simulink model "lccde2"  (Simulink 8.3)
settings: Solver=ode3  StartTime=0.0  StopTime=10.0  FixedStep=0.01  RelTol=1e-3
libraries: simulink x1
settings Model: Creator=Administrator  LastModifiedBy=Administrator
settings DataIOCC: SignalLoggingSaveFormat=Dataset
settings DebuggingCC: UnderspecifiedInitializationDetection=Simplified  StateNameClashWarn=none
settings GRTTargetCC: CombineOutputUpdateFcns=on  GRTInterface=off

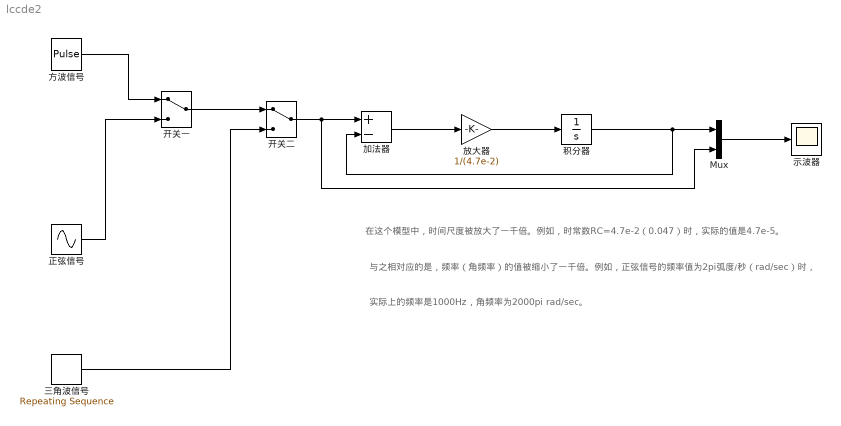
== system lccde2 ==
  note: 实际上的频率是1000Hz，角频率为2000pi rad/sec。
  note: 与之相对应的是，频率（角频率）的值被缩小了一千倍。例如，正弦信号的频率值为2pi弧度/秒（rad/sec）时，
  note: 在这个模型中，时间尺度被放大了一千倍。例如，时常数RC=4.7e-2（0.047）时，实际的值是4.7e-5。
  Mux : Mux  Inputs=2
  三角波信号 : simulink/Sources/Repeating Sequence  rep_seq_t=[0 0.5 1]  rep_seq_y=[0 2 0]
  加法器 : Sum  Inputs=+-
  开关一 : ManualSwitch
  开关二 : ManualSwitch
  放大器 : Gain  Gain=1/(4.7e-2)
  方波信号 : DiscretePulseGenerator  PulseType=Time based  Amplitude=3  Period=1  PulseWidth=50
  正弦信号 : Sin  Amplitude=3  Frequency=2*pi  SampleTime=0
  示波器 : Scope
  积分器 : Integrator
  wires:
  正弦信号/1 -> 开关一/2
  方波信号/1 -> 开关一/1
  加法器/1 -> 放大器/1
  放大器/1 -> 积分器/1
  积分器/1 -> Mux/1, 加法器/2
  Mux/1 -> 示波器/1
  三角波信号/1 -> 开关二/2
  开关一/1 -> 开关二/1
  开关二/1 -> Mux/2, 加法器/1
